simulink model "tennode_3"  (R2018b)
settings: Solver=ode3  StartTime=0.0  StopTime=5  FixedStep=Ts  RelTol=1e-3
values from neighbouring files (symbols this model uses):
  BESS_mode = 0    [load_vars.m]
  line1 = line1_length*R1    (= 0.01273)    [load_vars.m]
  line10 = line10_length*R1    (= 0.01273)    [load_vars.m]
  LINE10_en = 1    [load_vars.m]
  line11 = line11_length*R1    (= 0.01273)    [load_vars.m]
  LINE11_en = 1    [load_vars.m]
  line12 = line12_length*R1    (= 0.02546)    [load_vars.m]
  LINE12_en = 1    [load_vars.m]
  line13 = line13_length*R1    (= 0.015276)    [load_vars.m]
  LINE13_en = 1    [load_vars.m]
  line14 = line14_length*R1    (= 0.019095)    [load_vars.m]
  LINE14_en = 1    [load_vars.m]
  line15 = line15_length*R1    (= 0.014003)    [load_vars.m]
  LINE15_en = 1    [load_vars.m]
  line16 = line16_length*R1    (= 0.034371)    [load_vars.m]
  LINE16_en = 1    [load_vars.m]
  line17 = line17_length*R1    (= 0.017822)    [load_vars.m]
  LINE17_en = 1    [load_vars.m]
  LINE1_en = 1    [load_vars.m]
  line2 = line2_length*R1    (= 0.02546)    [load_vars.m]
  LINE2_en = 1    [load_vars.m]
  line3 = line3_length*R1    (= 0.015276)    [load_vars.m]
  LINE3_en = 1    [load_vars.m]
  line4 = line4_length*R1    (= 0.019095)    [load_vars.m]
  LINE4_en = 1    [load_vars.m]
  line5 = line5_length*R1    (= 0.014003)    [load_vars.m]
  LINE5_en = 1    [load_vars.m]
  line6 = line6_length*R1    (= 0.01273)    [load_vars.m]
  LINE6_en = 1    [load_vars.m]
  line7 = line7_length*R1    (= 0.03819)    [load_vars.m]
  LINE7_en = 1    [load_vars.m]
  line8 = line8_length*R1    (= 0.01273)    [load_vars.m]
  LINE8_en = 1    [load_vars.m]
  line9 = line9_length*R1    (= 0.01273)    [load_vars.m]
  LINE9_en = 1    [load_vars.m]
  t_contingency = 1    [load_vars.m]
  Ts = 0.0001    [load_vars.m]
  uDemand1 = 20e3    (= 20000)    [load_vars.m]
  uDemand10 = 20e3    (= 20000)    [load_vars.m]
  uDemand2 = 20e3    (= 20000)    [load_vars.m]
  uDemand3 = 20e3    (= 20000)    [load_vars.m]
  uDemand4 = 20e3    (= 20000)    [load_vars.m]
  uDemand5 = 20e3    (= 20000)    [load_vars.m]
  uDemand6 = 20e3    (= 20000)    [load_vars.m]
  uDemand7 = 20e3    (= 20000)    [load_vars.m]
  uDemand8 = 20e3    (= 20000)    [load_vars.m]
  uDemand9 = 20e3    (= 20000)    [load_vars.m]
undefined symbols (not defined in the file or in its folder): DER10_BESS_en, DER1_BESS_en, DER2_BESS_en, DER3_BESS_en, DER4_BESS_en, DER5_BESS_en, DER6_BESS_en, DER7_BESS_en, DER8_BESS_en, DER9_BESS_en, DR_capacity_1, DR_capacity_10, DR_capacity_2, DR_capacity_3, DR_capacity_4, DR_capacity_5, DR_capacity_6, DR_capacity_7, DR_capacity_8, DR_capacity_9, P_set1, P_set10, P_set2, P_set3, P_set4, P_set5, P_set6, P_set7, P_set8, P_set9, PV_capacity_1, PV_capacity_10, PV_capacity_2, PV_capacity_3, PV_capacity_4, PV_capacity_5, PV_capacity_6, PV_capacity_7, PV_capacity_8, PV_capacity_9, PV_en_1, PV_en_10, PV_en_2, PV_en_3, PV_en_4, PV_en_5, PV_en_6, PV_en_7, PV_en_8, PV_en_9
libraries: powerlib x232, simulink x66, powerlib_meascontrol x23, sps_avr x1, spsDieselMotorModel x1
(part 4 of 7)

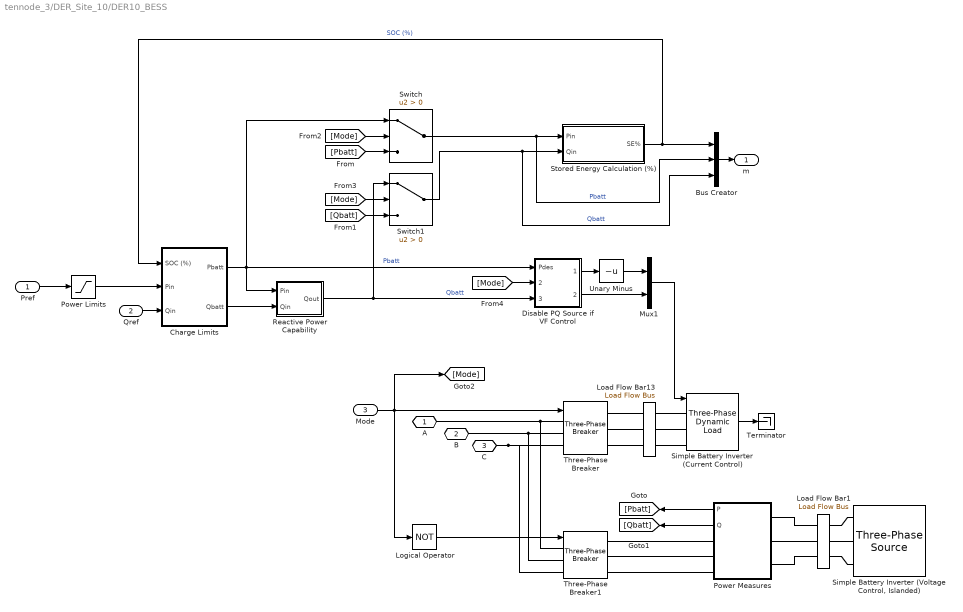
== system tennode_3/DER_Site_10/DER10_BESS ==
  Pref : Inport
  Qref : Inport  Port=2
  Mode : Inport  Port=3
  Bus Creator : BusCreator  Inputs=3
  Charge Limits : Subsystem
  Disable PQ Source if VF Control : Subsystem
  Load Flow Bar1 : powerlib/Measurements/Load Flow Bus  LConnTagsString=a|b|c  RConnTagsString=a|b|c  Phases=ABC  Connectors=on both sides  ID=5  Vbase=400/sqrt(3)  Vref=[1.0 1.0 1.0]  Vangle=[0 -120 120]  VLF=0.9823  VLFb=1.055  VLFc=0.9746  angleLF=-5.476  angleLFb=-122.5  angleLFc=116
      settings: AttributesFormatString=%<ID>  SourceProductName=Simscape Power Systems
  Load Flow Bar13 : powerlib/Measurements/Load Flow Bus  LConnTagsString=a|b|c  RConnTagsString=a|b|c  Phases=ABC  Connectors=on both sides  ID=4  Vbase=400/sqrt(3)  Vref=[1.0 1.0 1.0]  Vangle=[0 -120 120]  VLF=0.9823  VLFb=1.055  VLFc=0.9746  angleLF=-5.476  angleLFb=-122.5  angleLFc=116
      settings: AttributesFormatString=%<ID>  SourceProductName=Simscape Power Systems
  Logical Operator : Logic  Operator=NOT  AllPortsSameDT=off  OutDataTypeStr=boolean
  Mux1 : Mux  Inputs=2
  Power Limits : Saturate  UpperLimit=Pnom  LowerLimit=-Pnom
  Power Measures : Subsystem  VariantControlMode=Label  Variant=on  LabelModeActiveChoice=EMT
  Reactive Power Capability : Subsystem
  Simple Battery Inverter (Current Control) : powerlib/Elements/Three-Phase Dynamic Load  NominalVoltage=[Vn Fn]  ActiveReactivePowers=[-5000 -3.38813e-13]  PositiveSequence=[0.999844 -0.0038635]  ExternalControl=on  NpNq=[1.3 2]  TimeConstants="[0  0  0  0]"  MinimumVoltage=0.7  Tfilter=1e-2  LoadFlowParameters=[4,0,0,0,0]
      settings: SourceProductName=Simscape Electrical  SourceProductBaseCode=PS
  "Simple Battery Inverter (Voltage Control, Islanded)" : powerlib/Electrical Sources/Three-Phase Source  InternalConnection=Yg  VoltagePhases=off  Voltage=Vn  PhaseAngle=0  Voltage_phases=[25e3 25e3 25e3]/sqrt(3)  PhaseAngles_phases=[0 -120 +120]  Frequency=Fn  NonIdealSource=off  SpecifyImpedance=off  Resistance=0.8929  Inductance=16.58e-3  ShortCircuitLevel=100e6  BaseVoltage=25e3  XRratio=7  BusType=swing  Pref=10e3  Qref=0  Prefabc=[10e3, 10e3, 10e3]  Qrefabc=[0, 0, 0]  Qmin=-inf  Qmax=inf
      settings: SourceProductName=Simscape Electrical
  Stored Energy Calculation (%) : Subsystem
  Switch : Switch  Criteria=u2 > Threshold
  Switch1 : Switch  Criteria=u2 > Threshold
  Terminator : Terminator
  Three-Phase Breaker : powerlib/Elements/Three-Phase Breaker  InitialState=closed  SwitchA=on  SwitchB=on  SwitchC=on  SwitchTimes="[1/60  5/60]"  External=on  BreakerResistance=0.01  SnubberResistance=1e6  SnubberCapacitance=inf  Measurements=None
      settings: SourceProductName=Simscape Electrical
  Three-Phase Breaker1 : powerlib/Elements/Three-Phase Breaker  InitialState=open  SwitchA=on  SwitchB=on  SwitchC=on  SwitchTimes="[1/60  5/60]"  External=on  BreakerResistance=0.01  SnubberResistance=1e6  SnubberCapacitance=inf  Measurements=None
      settings: SourceProductName=Simscape Electrical
  Unary Minus : UnaryMinus
  A : PMIOPort  Side=Right
  B : PMIOPort  Port=2  Side=Right
  C : PMIOPort  Port=3  Side=Right
  m : Outport
  wires:
  Disable PQ Source if VF Control/2(Qbatt) -> Mux1/2
  Disable PQ Source if VF Control/1(Pbatt) -> Unary Minus/1
  Reactive Power Capability/1(Qout) -> Switch1/1, Disable PQ Source if VF Control/3(Qdes)  "Qbatt"
  [Mode] -> Disable PQ Source if VF Control/2(Mode)
  Charge Limits/1(Pbatt) -> Disable PQ Source if VF Control/1(Pdes), Reactive Power Capability/1(Pin), Switch/1  "Pbatt"
  [Pbatt] -> Switch/3
  [Qbatt] -> Switch1/3
  [Mode] -> Switch1/2
  [Mode] -> Switch/2
  Switch1/1 -> Stored Energy Calculation (%)/2(Qin), Bus Creator/3  "Qbatt"
  Switch/1 -> Stored Energy Calculation (%)/1(Pin), Bus Creator/2  "Pbatt"
  Power Measures/2(Q) -> [Qbatt]
  Power Measures/1(P) -> [Pbatt]
  Mode/1 -> Three-Phase Breaker/1, Logical Operator/1, [Mode]
  Logical Operator/1 -> Three-Phase Breaker1/1
  Unary Minus/1 -> Mux1/1
  Mux1/1 -> Simple Battery Inverter (Current Control)/1
  Simple Battery Inverter (Current Control)/1 -> Terminator/1
  Pref/1 -> Power Limits/1
  Bus Creator/1 -> m/1
  Stored Energy Calculation (%)/1(SE%) -> Charge Limits/1(SOC (%)), Bus Creator/1  "SOC (%)"
  Power Limits/1 -> Charge Limits/2(Pin)
  Qref/1 -> Charge Limits/3(Qin)
  Charge Limits/2(Qbatt) -> Reactive Power Capability/2(Qin)
  connections:
  Power Measures/RConn3 -- Three-Phase Breaker1/RConn3
  Power Measures/RConn2 -- Three-Phase Breaker1/RConn2
  Power Measures/RConn1 -- Three-Phase Breaker1/RConn1
  Three-Phase Breaker1/LConn1 -- A/RConn1 -- Three-Phase Breaker/LConn1
  Three-Phase Breaker1/LConn2 -- B/RConn1 -- Three-Phase Breaker/LConn2
  C/RConn1 -- Three-Phase Breaker1/LConn3 -- Three-Phase Breaker/LConn3
  Load Flow Bar13/RConn1 -- Three-Phase Breaker/RConn1
  Load Flow Bar13/RConn2 -- Three-Phase Breaker/RConn2
  Load Flow Bar13/RConn3 -- Three-Phase Breaker/RConn3
  Load Flow Bar13/LConn1 -- Simple Battery Inverter (Current Control)/LConn1
  Load Flow Bar13/LConn2 -- Simple Battery Inverter (Current Control)/LConn2
  Load Flow Bar13/LConn3 -- Simple Battery Inverter (Current Control)/LConn3
  "Simple Battery Inverter (Voltage Control, Islanded)"/RConn2 -- Load Flow Bar1/LConn2
  Load Flow Bar1/LConn3 -- "Simple Battery Inverter (Voltage Control, Islanded)"/RConn3
  Load Flow Bar1/LConn1 -- "Simple Battery Inverter (Voltage Control, Islanded)"/RConn1
  Power Measures/LConn1 -- Load Flow Bar1/RConn1
  Power Measures/LConn2 -- Load Flow Bar1/RConn2
  Power Measures/LConn3 -- Load Flow Bar1/RConn3

== system tennode_3/DER_Site_10/DER10_PV  ==
  P : Inport
  Bus Selector : BusSelector  OutputSignals=Active power P (W)
  Constant11 : Constant  Value=0
  Mux1 : Mux  Inputs=2
  Simple Solar Inverter : powerlib/Elements/Three-Phase Dynamic Load  NominalVoltage=[Vn Fn]  ActiveReactivePowers=[-4000 -3.38813e-13]  PositiveSequence=[0.999844 -0.0038635]  ExternalControl=on  NpNq=[1.3 2]  TimeConstants="[0  0  0  0]"  MinimumVoltage=0.7  Tfilter=1e-2  LoadFlowParameters=[4,0,0,0,0]
      settings: SourceProductName=Simscape Electrical  SourceProductBaseCode=PS
  Unary Minus : UnaryMinus
  Unary Minus1 : UnaryMinus
  A : PMIOPort  Side=Right
  B : PMIOPort  Port=2  Side=Right
  C : PMIOPort  Port=3  Side=Right
  m : Outport
  wires:
  P/1 -> Unary Minus/1
  Unary Minus/1 -> Mux1/1
  Mux1/1 -> Simple Solar Inverter/1
  Constant11/1 -> Mux1/2
  Simple Solar Inverter/1 -> Bus Selector/1
  Bus Selector/1 -> Unary Minus1/1  "<Active power P (W)>"
  Unary Minus1/1 -> m/1
  connections:
  Simple Solar Inverter/LConn2 -- B/RConn1
  Simple Solar Inverter/LConn3 -- C/RConn1
  Simple Solar Inverter/LConn1 -- A/RConn1

== system tennode_3/DER_Site_10/Site Load ==
  Load : Inport
  Dynamic Load Control : Subsystem
  Simple Three-Phase Load : powerlib/Elements/Three-Phase Dynamic Load  NominalVoltage=[Vn Fn]  ActiveReactivePowers=[200000 45883.1]  PositiveSequence=[0.999844 -0.0038635]  ExternalControl=on  NpNq=[1.3 2]  TimeConstants="[0  0  0  0]"  MinimumVoltage=0.7  Tfilter=1e-2  LoadFlowParameters=[4,0,0,0,0]
      settings: SourceProductName=Simscape Electrical  SourceProductBaseCode=PS
  A : PMIOPort  Side=Right
  B : PMIOPort  Port=2  Side=Right
  C : PMIOPort  Port=3  Side=Right
  m : Outport
  wires:
  Load/1 -> Dynamic Load Control/1(P0)
  Dynamic Load Control/1(PQ) -> Simple Three-Phase Load/1
  Simple Three-Phase Load/1 -> m/1
  connections:
  Simple Three-Phase Load/LConn1 -- A/RConn1
  Simple Three-Phase Load/LConn3 -- C/RConn1
  Simple Three-Phase Load/LConn2 -- B/RConn1

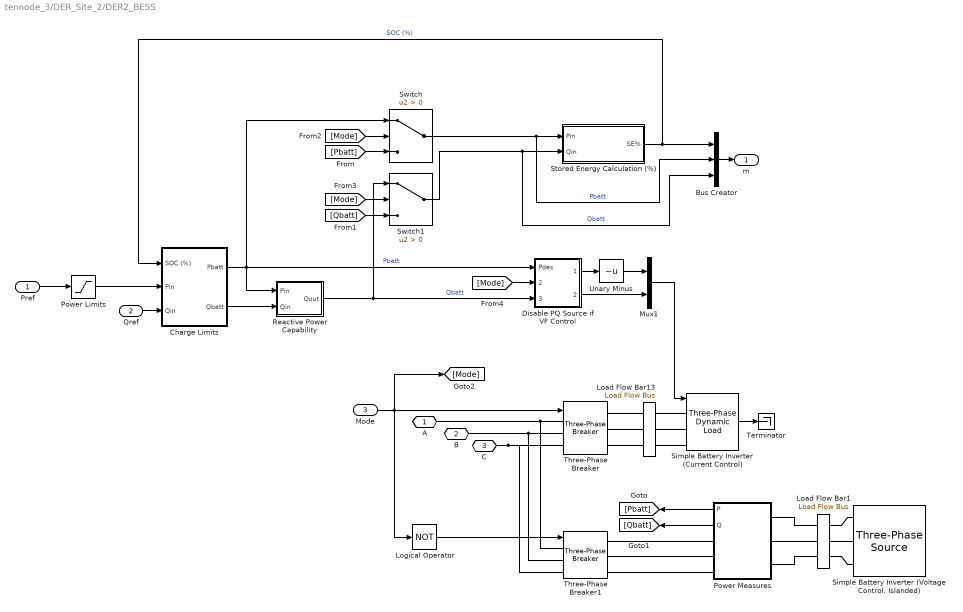
== system tennode_3/DER_Site_2/DER2_BESS ==
  Pref : Inport
  Qref : Inport  Port=2
  Mode : Inport  Port=3
  Bus Creator : BusCreator  Inputs=3
  Charge Limits : Subsystem
  Disable PQ Source if VF Control : Subsystem
  Load Flow Bar1 : powerlib/Measurements/Load Flow Bus  LConnTagsString=a|b|c  RConnTagsString=a|b|c  Phases=ABC  Connectors=on both sides  ID=5  Vbase=400/sqrt(3)  Vref=[1.0 1.0 1.0]  Vangle=[0 -120 120]  VLF=0.9823  VLFb=1.055  VLFc=0.9746  angleLF=-5.476  angleLFb=-122.5  angleLFc=116
      settings: AttributesFormatString=%<ID>  SourceProductName=Simscape Power Systems
  Load Flow Bar13 : powerlib/Measurements/Load Flow Bus  LConnTagsString=a|b|c  RConnTagsString=a|b|c  Phases=ABC  Connectors=on both sides  ID=4  Vbase=400/sqrt(3)  Vref=[1.0 1.0 1.0]  Vangle=[0 -120 120]  VLF=0.9823  VLFb=1.055  VLFc=0.9746  angleLF=-5.476  angleLFb=-122.5  angleLFc=116
      settings: AttributesFormatString=%<ID>  SourceProductName=Simscape Power Systems
  Logical Operator : Logic  Operator=NOT  AllPortsSameDT=off  OutDataTypeStr=boolean
  Mux1 : Mux  Inputs=2
  Power Limits : Saturate  UpperLimit=Pnom  LowerLimit=-Pnom
  Power Measures : Subsystem  VariantControlMode=Label  Variant=on  LabelModeActiveChoice=EMT
  Reactive Power Capability : Subsystem
  Simple Battery Inverter (Current Control) : powerlib/Elements/Three-Phase Dynamic Load  NominalVoltage=[Vn Fn]  ActiveReactivePowers=[-5000 -3.38813e-13]  PositiveSequence=[0.999844 -0.0038635]  ExternalControl=on  NpNq=[1.3 2]  TimeConstants="[0  0  0  0]"  MinimumVoltage=0.7  Tfilter=1e-2  LoadFlowParameters=[4,0,0,0,0]
      settings: SourceProductName=Simscape Electrical  SourceProductBaseCode=PS
  "Simple Battery Inverter (Voltage Control, Islanded)" : powerlib/Electrical Sources/Three-Phase Source  InternalConnection=Yg  VoltagePhases=off  Voltage=Vn  PhaseAngle=0  Voltage_phases=[25e3 25e3 25e3]/sqrt(3)  PhaseAngles_phases=[0 -120 +120]  Frequency=Fn  NonIdealSource=off  SpecifyImpedance=off  Resistance=0.8929  Inductance=16.58e-3  ShortCircuitLevel=100e6  BaseVoltage=25e3  XRratio=7  BusType=swing  Pref=10e3  Qref=0  Prefabc=[10e3, 10e3, 10e3]  Qrefabc=[0, 0, 0]  Qmin=-inf  Qmax=inf
      settings: SourceProductName=Simscape Electrical
  Stored Energy Calculation (%) : Subsystem
  Switch : Switch  Criteria=u2 > Threshold
  Switch1 : Switch  Criteria=u2 > Threshold
  Terminator : Terminator
  Three-Phase Breaker : powerlib/Elements/Three-Phase Breaker  InitialState=closed  SwitchA=on  SwitchB=on  SwitchC=on  SwitchTimes="[1/60  5/60]"  External=on  BreakerResistance=0.01  SnubberResistance=1e6  SnubberCapacitance=inf  Measurements=None
      settings: SourceProductName=Simscape Electrical
  Three-Phase Breaker1 : powerlib/Elements/Three-Phase Breaker  InitialState=open  SwitchA=on  SwitchB=on  SwitchC=on  SwitchTimes="[1/60  5/60]"  External=on  BreakerResistance=0.01  SnubberResistance=1e6  SnubberCapacitance=inf  Measurements=None
      settings: SourceProductName=Simscape Electrical
  Unary Minus : UnaryMinus
  A : PMIOPort  Side=Right
  B : PMIOPort  Port=2  Side=Right
  C : PMIOPort  Port=3  Side=Right
  m : Outport
  wires:
  Disable PQ Source if VF Control/2(Qbatt) -> Mux1/2
  Disable PQ Source if VF Control/1(Pbatt) -> Unary Minus/1
  Reactive Power Capability/1(Qout) -> Switch1/1, Disable PQ Source if VF Control/3(Qdes)  "Qbatt"
  [Mode] -> Disable PQ Source if VF Control/2(Mode)
  Charge Limits/1(Pbatt) -> Disable PQ Source if VF Control/1(Pdes), Reactive Power Capability/1(Pin), Switch/1  "Pbatt"
  [Pbatt] -> Switch/3
  [Qbatt] -> Switch1/3
  [Mode] -> Switch1/2
  [Mode] -> Switch/2
  Switch1/1 -> Stored Energy Calculation (%)/2(Qin), Bus Creator/3  "Qbatt"
  Switch/1 -> Stored Energy Calculation (%)/1(Pin), Bus Creator/2  "Pbatt"
  Power Measures/2(Q) -> [Qbatt]
  Power Measures/1(P) -> [Pbatt]
  Mode/1 -> Three-Phase Breaker/1, Logical Operator/1, [Mode]
  Logical Operator/1 -> Three-Phase Breaker1/1
  Unary Minus/1 -> Mux1/1
  Mux1/1 -> Simple Battery Inverter (Current Control)/1
  Simple Battery Inverter (Current Control)/1 -> Terminator/1
  Pref/1 -> Power Limits/1
  Bus Creator/1 -> m/1
  Stored Energy Calculation (%)/1(SE%) -> Charge Limits/1(SOC (%)), Bus Creator/1  "SOC (%)"
  Power Limits/1 -> Charge Limits/2(Pin)
  Qref/1 -> Charge Limits/3(Qin)
  Charge Limits/2(Qbatt) -> Reactive Power Capability/2(Qin)
  connections:
  Power Measures/RConn3 -- Three-Phase Breaker1/RConn3
  Power Measures/RConn2 -- Three-Phase Breaker1/RConn2
  Power Measures/RConn1 -- Three-Phase Breaker1/RConn1
  Three-Phase Breaker1/LConn1 -- A/RConn1 -- Three-Phase Breaker/LConn1
  Three-Phase Breaker1/LConn2 -- B/RConn1 -- Three-Phase Breaker/LConn2
  C/RConn1 -- Three-Phase Breaker1/LConn3 -- Three-Phase Breaker/LConn3
  Load Flow Bar13/RConn1 -- Three-Phase Breaker/RConn1
  Load Flow Bar13/RConn2 -- Three-Phase Breaker/RConn2
  Load Flow Bar13/RConn3 -- Three-Phase Breaker/RConn3
  Load Flow Bar13/LConn1 -- Simple Battery Inverter (Current Control)/LConn1
  Load Flow Bar13/LConn2 -- Simple Battery Inverter (Current Control)/LConn2
  Load Flow Bar13/LConn3 -- Simple Battery Inverter (Current Control)/LConn3
  "Simple Battery Inverter (Voltage Control, Islanded)"/RConn2 -- Load Flow Bar1/LConn2
  Load Flow Bar1/LConn3 -- "Simple Battery Inverter (Voltage Control, Islanded)"/RConn3
  Load Flow Bar1/LConn1 -- "Simple Battery Inverter (Voltage Control, Islanded)"/RConn1
  Power Measures/LConn1 -- Load Flow Bar1/RConn1
  Power Measures/LConn2 -- Load Flow Bar1/RConn2
  Power Measures/LConn3 -- Load Flow Bar1/RConn3

== system tennode_3/DER_Site_2/DER2_PV  ==
  P : Inport
  Bus Selector : BusSelector  OutputSignals=Active power P (W)
  Constant11 : Constant  Value=0
  Mux1 : Mux  Inputs=2
  Simple Solar Inverter : powerlib/Elements/Three-Phase Dynamic Load  NominalVoltage=[Vn Fn]  ActiveReactivePowers=[-4000 -3.38813e-13]  PositiveSequence=[0.999844 -0.0038635]  ExternalControl=on  NpNq=[1.3 2]  TimeConstants="[0  0  0  0]"  MinimumVoltage=0.7  Tfilter=1e-2  LoadFlowParameters=[4,0,0,0,0]
      settings: SourceProductName=Simscape Electrical  SourceProductBaseCode=PS
  Unary Minus : UnaryMinus
  Unary Minus1 : UnaryMinus
  A : PMIOPort  Side=Right
  B : PMIOPort  Port=2  Side=Right
  C : PMIOPort  Port=3  Side=Right
  m : Outport
  wires:
  P/1 -> Unary Minus/1
  Unary Minus/1 -> Mux1/1
  Mux1/1 -> Simple Solar Inverter/1
  Constant11/1 -> Mux1/2
  Simple Solar Inverter/1 -> Bus Selector/1
  Bus Selector/1 -> Unary Minus1/1  "<Active power P (W)>"
  Unary Minus1/1 -> m/1
  connections:
  Simple Solar Inverter/LConn2 -- B/RConn1
  Simple Solar Inverter/LConn3 -- C/RConn1
  Simple Solar Inverter/LConn1 -- A/RConn1

== system tennode_3/DER_Site_2/Site Load ==
  Load : Inport
  Dynamic Load Control : Subsystem
  Simple Three-Phase Load : powerlib/Elements/Three-Phase Dynamic Load  NominalVoltage=[Vn Fn]  ActiveReactivePowers=[200000 45883.1]  PositiveSequence=[0.999844 -0.0038635]  ExternalControl=on  NpNq=[1.3 2]  TimeConstants="[0  0  0  0]"  MinimumVoltage=0.7  Tfilter=1e-2  LoadFlowParameters=[4,0,0,0,0]
      settings: SourceProductName=Simscape Electrical  SourceProductBaseCode=PS
  A : PMIOPort  Side=Right
  B : PMIOPort  Port=2  Side=Right
  C : PMIOPort  Port=3  Side=Right
  m : Outport
  wires:
  Load/1 -> Dynamic Load Control/1(P0)
  Dynamic Load Control/1(PQ) -> Simple Three-Phase Load/1
  Simple Three-Phase Load/1 -> m/1
  connections:
  Simple Three-Phase Load/LConn1 -- A/RConn1
  Simple Three-Phase Load/LConn3 -- C/RConn1
  Simple Three-Phase Load/LConn2 -- B/RConn1

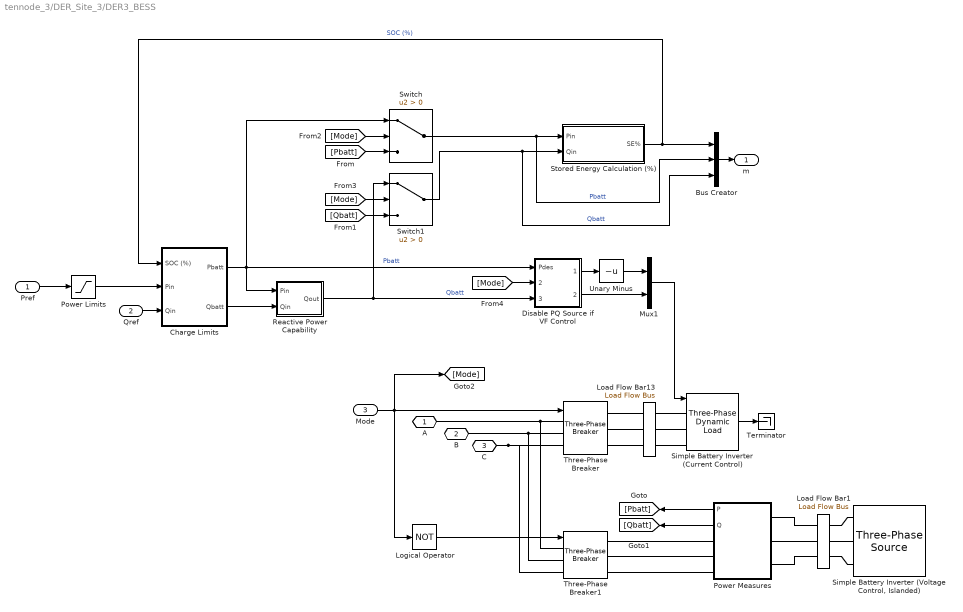
== system tennode_3/DER_Site_3/DER3_BESS ==
  Pref : Inport
  Qref : Inport  Port=2
  Mode : Inport  Port=3
  Bus Creator : BusCreator  Inputs=3
  Charge Limits : Subsystem
  Disable PQ Source if VF Control : Subsystem
  Load Flow Bar1 : powerlib/Measurements/Load Flow Bus  LConnTagsString=a|b|c  RConnTagsString=a|b|c  Phases=ABC  Connectors=on both sides  ID=5  Vbase=400/sqrt(3)  Vref=[1.0 1.0 1.0]  Vangle=[0 -120 120]  VLF=0.9823  VLFb=1.055  VLFc=0.9746  angleLF=-5.476  angleLFb=-122.5  angleLFc=116
      settings: AttributesFormatString=%<ID>  SourceProductName=Simscape Power Systems
  Load Flow Bar13 : powerlib/Measurements/Load Flow Bus  LConnTagsString=a|b|c  RConnTagsString=a|b|c  Phases=ABC  Connectors=on both sides  ID=4  Vbase=400/sqrt(3)  Vref=[1.0 1.0 1.0]  Vangle=[0 -120 120]  VLF=0.9823  VLFb=1.055  VLFc=0.9746  angleLF=-5.476  angleLFb=-122.5  angleLFc=116
      settings: AttributesFormatString=%<ID>  SourceProductName=Simscape Power Systems
  Logical Operator : Logic  Operator=NOT  AllPortsSameDT=off  OutDataTypeStr=boolean
  Mux1 : Mux  Inputs=2
  Power Limits : Saturate  UpperLimit=Pnom  LowerLimit=-Pnom
  Power Measures : Subsystem  VariantControlMode=Label  Variant=on  LabelModeActiveChoice=EMT
  Reactive Power Capability : Subsystem
  Simple Battery Inverter (Current Control) : powerlib/Elements/Three-Phase Dynamic Load  NominalVoltage=[Vn Fn]  ActiveReactivePowers=[-5000 -3.38813e-13]  PositiveSequence=[0.999844 -0.0038635]  ExternalControl=on  NpNq=[1.3 2]  TimeConstants="[0  0  0  0]"  MinimumVoltage=0.7  Tfilter=1e-2  LoadFlowParameters=[4,0,0,0,0]
      settings: SourceProductName=Simscape Electrical  SourceProductBaseCode=PS
  "Simple Battery Inverter (Voltage Control, Islanded)" : powerlib/Electrical Sources/Three-Phase Source  InternalConnection=Yg  VoltagePhases=off  Voltage=Vn  PhaseAngle=0  Voltage_phases=[25e3 25e3 25e3]/sqrt(3)  PhaseAngles_phases=[0 -120 +120]  Frequency=Fn  NonIdealSource=off  SpecifyImpedance=off  Resistance=0.8929  Inductance=16.58e-3  ShortCircuitLevel=100e6  BaseVoltage=25e3  XRratio=7  BusType=swing  Pref=10e3  Qref=0  Prefabc=[10e3, 10e3, 10e3]  Qrefabc=[0, 0, 0]  Qmin=-inf  Qmax=inf
      settings: SourceProductName=Simscape Electrical
  Stored Energy Calculation (%) : Subsystem
  Switch : Switch  Criteria=u2 > Threshold
  Switch1 : Switch  Criteria=u2 > Threshold
  Terminator : Terminator
  Three-Phase Breaker : powerlib/Elements/Three-Phase Breaker  InitialState=closed  SwitchA=on  SwitchB=on  SwitchC=on  SwitchTimes="[1/60  5/60]"  External=on  BreakerResistance=0.01  SnubberResistance=1e6  SnubberCapacitance=inf  Measurements=None
      settings: SourceProductName=Simscape Electrical
  Three-Phase Breaker1 : powerlib/Elements/Three-Phase Breaker  InitialState=open  SwitchA=on  SwitchB=on  SwitchC=on  SwitchTimes="[1/60  5/60]"  External=on  BreakerResistance=0.01  SnubberResistance=1e6  SnubberCapacitance=inf  Measurements=None
      settings: SourceProductName=Simscape Electrical
  Unary Minus : UnaryMinus
  A : PMIOPort  Side=Right
  B : PMIOPort  Port=2  Side=Right
  C : PMIOPort  Port=3  Side=Right
  m : Outport
  wires:
  Disable PQ Source if VF Control/2(Qbatt) -> Mux1/2
  Disable PQ Source if VF Control/1(Pbatt) -> Unary Minus/1
  Reactive Power Capability/1(Qout) -> Switch1/1, Disable PQ Source if VF Control/3(Qdes)  "Qbatt"
  [Mode] -> Disable PQ Source if VF Control/2(Mode)
  Charge Limits/1(Pbatt) -> Disable PQ Source if VF Control/1(Pdes), Reactive Power Capability/1(Pin), Switch/1  "Pbatt"
  [Pbatt] -> Switch/3
  [Qbatt] -> Switch1/3
  [Mode] -> Switch1/2
  [Mode] -> Switch/2
  Switch1/1 -> Stored Energy Calculation (%)/2(Qin), Bus Creator/3  "Qbatt"
  Switch/1 -> Stored Energy Calculation (%)/1(Pin), Bus Creator/2  "Pbatt"
  Power Measures/2(Q) -> [Qbatt]
  Power Measures/1(P) -> [Pbatt]
  Mode/1 -> Three-Phase Breaker/1, Logical Operator/1, [Mode]
  Logical Operator/1 -> Three-Phase Breaker1/1
  Unary Minus/1 -> Mux1/1
  Mux1/1 -> Simple Battery Inverter (Current Control)/1
  Simple Battery Inverter (Current Control)/1 -> Terminator/1
  Pref/1 -> Power Limits/1
  Bus Creator/1 -> m/1
  Stored Energy Calculation (%)/1(SE%) -> Charge Limits/1(SOC (%)), Bus Creator/1  "SOC (%)"
  Power Limits/1 -> Charge Limits/2(Pin)
  Qref/1 -> Charge Limits/3(Qin)
  Charge Limits/2(Qbatt) -> Reactive Power Capability/2(Qin)
  connections:
  Power Measures/RConn3 -- Three-Phase Breaker1/RConn3
  Power Measures/RConn2 -- Three-Phase Breaker1/RConn2
  Power Measures/RConn1 -- Three-Phase Breaker1/RConn1
  Three-Phase Breaker1/LConn1 -- A/RConn1 -- Three-Phase Breaker/LConn1
  Three-Phase Breaker1/LConn2 -- B/RConn1 -- Three-Phase Breaker/LConn2
  C/RConn1 -- Three-Phase Breaker1/LConn3 -- Three-Phase Breaker/LConn3
  Load Flow Bar13/RConn1 -- Three-Phase Breaker/RConn1
  Load Flow Bar13/RConn2 -- Three-Phase Breaker/RConn2
  Load Flow Bar13/RConn3 -- Three-Phase Breaker/RConn3
  Load Flow Bar13/LConn1 -- Simple Battery Inverter (Current Control)/LConn1
  Load Flow Bar13/LConn2 -- Simple Battery Inverter (Current Control)/LConn2
  Load Flow Bar13/LConn3 -- Simple Battery Inverter (Current Control)/LConn3
  "Simple Battery Inverter (Voltage Control, Islanded)"/RConn2 -- Load Flow Bar1/LConn2
  Load Flow Bar1/LConn3 -- "Simple Battery Inverter (Voltage Control, Islanded)"/RConn3
  Load Flow Bar1/LConn1 -- "Simple Battery Inverter (Voltage Control, Islanded)"/RConn1
  Power Measures/LConn1 -- Load Flow Bar1/RConn1
  Power Measures/LConn2 -- Load Flow Bar1/RConn2
  Power Measures/LConn3 -- Load Flow Bar1/RConn3

== system tennode_3/DER_Site_3/DER3_PV  ==
  P : Inport
  Bus Selector : BusSelector  OutputSignals=Active power P (W)
  Constant11 : Constant  Value=0
  Mux1 : Mux  Inputs=2
  Simple Solar Inverter : powerlib/Elements/Three-Phase Dynamic Load  NominalVoltage=[Vn Fn]  ActiveReactivePowers=[-4000 -3.38813e-13]  PositiveSequence=[0.999844 -0.0038635]  ExternalControl=on  NpNq=[1.3 2]  TimeConstants="[0  0  0  0]"  MinimumVoltage=0.7  Tfilter=1e-2  LoadFlowParameters=[4,0,0,0,0]
      settings: SourceProductName=Simscape Electrical  SourceProductBaseCode=PS
  Unary Minus : UnaryMinus
  Unary Minus1 : UnaryMinus
  A : PMIOPort  Side=Right
  B : PMIOPort  Port=2  Side=Right
  C : PMIOPort  Port=3  Side=Right
  m : Outport
  wires:
  P/1 -> Unary Minus/1
  Unary Minus/1 -> Mux1/1
  Mux1/1 -> Simple Solar Inverter/1
  Constant11/1 -> Mux1/2
  Simple Solar Inverter/1 -> Bus Selector/1
  Bus Selector/1 -> Unary Minus1/1  "<Active power P (W)>"
  Unary Minus1/1 -> m/1
  connections:
  Simple Solar Inverter/LConn2 -- B/RConn1
  Simple Solar Inverter/LConn3 -- C/RConn1
  Simple Solar Inverter/LConn1 -- A/RConn1

== system tennode_3/DER_Site_3/Site Load ==
  Load : Inport
  Dynamic Load Control : Subsystem
  Simple Three-Phase Load : powerlib/Elements/Three-Phase Dynamic Load  NominalVoltage=[Vn Fn]  ActiveReactivePowers=[200000 45883.1]  PositiveSequence=[0.999844 -0.0038635]  ExternalControl=on  NpNq=[1.3 2]  TimeConstants="[0  0  0  0]"  MinimumVoltage=0.7  Tfilter=1e-2  LoadFlowParameters=[4,0,0,0,0]
      settings: SourceProductName=Simscape Electrical  SourceProductBaseCode=PS
  A : PMIOPort  Side=Right
  B : PMIOPort  Port=2  Side=Right
  C : PMIOPort  Port=3  Side=Right
  m : Outport
  wires:
  Load/1 -> Dynamic Load Control/1(P0)
  Dynamic Load Control/1(PQ) -> Simple Three-Phase Load/1
  Simple Three-Phase Load/1 -> m/1
  connections:
  Simple Three-Phase Load/LConn1 -- A/RConn1
  Simple Three-Phase Load/LConn3 -- C/RConn1
  Simple Three-Phase Load/LConn2 -- B/RConn1

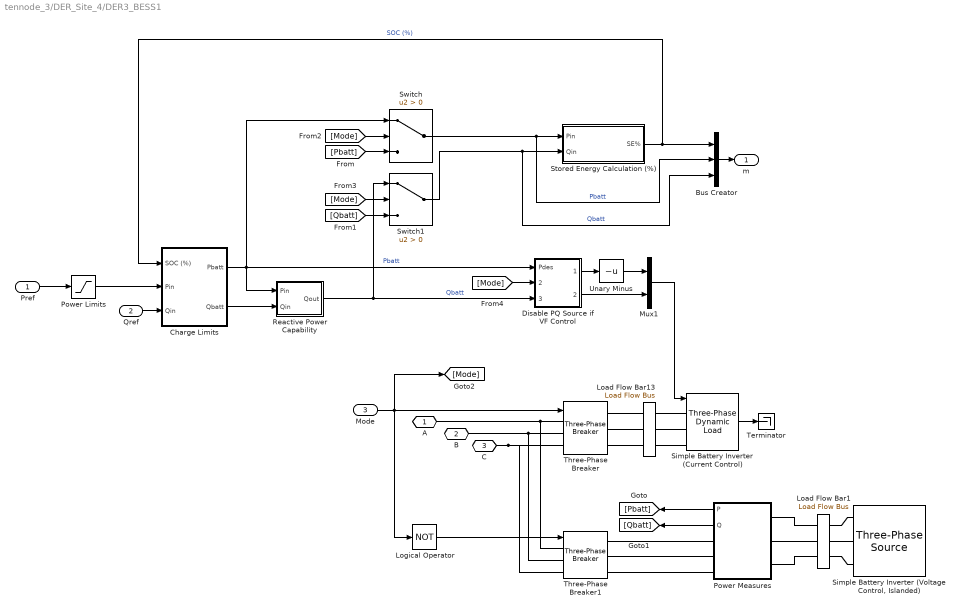
== system tennode_3/DER_Site_4/DER3_BESS1 ==
  Pref : Inport
  Qref : Inport  Port=2
  Mode : Inport  Port=3
  Bus Creator : BusCreator  Inputs=3
  Charge Limits : Subsystem
  Disable PQ Source if VF Control : Subsystem
  Load Flow Bar1 : powerlib/Measurements/Load Flow Bus  LConnTagsString=a|b|c  RConnTagsString=a|b|c  Phases=ABC  Connectors=on both sides  ID=5  Vbase=400/sqrt(3)  Vref=[1.0 1.0 1.0]  Vangle=[0 -120 120]  VLF=0.9823  VLFb=1.055  VLFc=0.9746  angleLF=-5.476  angleLFb=-122.5  angleLFc=116
      settings: AttributesFormatString=%<ID>  SourceProductName=Simscape Power Systems
  Load Flow Bar13 : powerlib/Measurements/Load Flow Bus  LConnTagsString=a|b|c  RConnTagsString=a|b|c  Phases=ABC  Connectors=on both sides  ID=4  Vbase=400/sqrt(3)  Vref=[1.0 1.0 1.0]  Vangle=[0 -120 120]  VLF=0.9823  VLFb=1.055  VLFc=0.9746  angleLF=-5.476  angleLFb=-122.5  angleLFc=116
      settings: AttributesFormatString=%<ID>  SourceProductName=Simscape Power Systems
  Logical Operator : Logic  Operator=NOT  AllPortsSameDT=off  OutDataTypeStr=boolean
  Mux1 : Mux  Inputs=2
  Power Limits : Saturate  UpperLimit=Pnom  LowerLimit=-Pnom
  Power Measures : Subsystem  VariantControlMode=Label  Variant=on  LabelModeActiveChoice=EMT
  Reactive Power Capability : Subsystem
  Simple Battery Inverter (Current Control) : powerlib/Elements/Three-Phase Dynamic Load  NominalVoltage=[Vn Fn]  ActiveReactivePowers=[-5000 -3.38813e-13]  PositiveSequence=[0.999844 -0.0038635]  ExternalControl=on  NpNq=[1.3 2]  TimeConstants="[0  0  0  0]"  MinimumVoltage=0.7  Tfilter=1e-2  LoadFlowParameters=[4,0,0,0,0]
      settings: SourceProductName=Simscape Electrical  SourceProductBaseCode=PS
  "Simple Battery Inverter (Voltage Control, Islanded)" : powerlib/Electrical Sources/Three-Phase Source  InternalConnection=Yg  VoltagePhases=off  Voltage=Vn  PhaseAngle=0  Voltage_phases=[25e3 25e3 25e3]/sqrt(3)  PhaseAngles_phases=[0 -120 +120]  Frequency=Fn  NonIdealSource=off  SpecifyImpedance=off  Resistance=0.8929  Inductance=16.58e-3  ShortCircuitLevel=100e6  BaseVoltage=25e3  XRratio=7  BusType=swing  Pref=10e3  Qref=0  Prefabc=[10e3, 10e3, 10e3]  Qrefabc=[0, 0, 0]  Qmin=-inf  Qmax=inf
      settings: SourceProductName=Simscape Electrical
  Stored Energy Calculation (%) : Subsystem
  Switch : Switch  Criteria=u2 > Threshold
  Switch1 : Switch  Criteria=u2 > Threshold
  Terminator : Terminator
  Three-Phase Breaker : powerlib/Elements/Three-Phase Breaker  InitialState=closed  SwitchA=on  SwitchB=on  SwitchC=on  SwitchTimes="[1/60  5/60]"  External=on  BreakerResistance=0.01  SnubberResistance=1e6  SnubberCapacitance=inf  Measurements=None
      settings: SourceProductName=Simscape Electrical
  Three-Phase Breaker1 : powerlib/Elements/Three-Phase Breaker  InitialState=open  SwitchA=on  SwitchB=on  SwitchC=on  SwitchTimes="[1/60  5/60]"  External=on  BreakerResistance=0.01  SnubberResistance=1e6  SnubberCapacitance=inf  Measurements=None
      settings: SourceProductName=Simscape Electrical
  Unary Minus : UnaryMinus
  A : PMIOPort  Side=Right
  B : PMIOPort  Port=2  Side=Right
  C : PMIOPort  Port=3  Side=Right
  m : Outport
  wires:
  Disable PQ Source if VF Control/2(Qbatt) -> Mux1/2
  Disable PQ Source if VF Control/1(Pbatt) -> Unary Minus/1
  Reactive Power Capability/1(Qout) -> Switch1/1, Disable PQ Source if VF Control/3(Qdes)  "Qbatt"
  [Mode] -> Disable PQ Source if VF Control/2(Mode)
  Charge Limits/1(Pbatt) -> Disable PQ Source if VF Control/1(Pdes), Reactive Power Capability/1(Pin), Switch/1  "Pbatt"
  [Pbatt] -> Switch/3
  [Qbatt] -> Switch1/3
  [Mode] -> Switch1/2
  [Mode] -> Switch/2
  Switch1/1 -> Stored Energy Calculation (%)/2(Qin), Bus Creator/3  "Qbatt"
  Switch/1 -> Stored Energy Calculation (%)/1(Pin), Bus Creator/2  "Pbatt"
  Power Measures/2(Q) -> [Qbatt]
  Power Measures/1(P) -> [Pbatt]
  Mode/1 -> Three-Phase Breaker/1, Logical Operator/1, [Mode]
  Logical Operator/1 -> Three-Phase Breaker1/1
  Unary Minus/1 -> Mux1/1
  Mux1/1 -> Simple Battery Inverter (Current Control)/1
  Simple Battery Inverter (Current Control)/1 -> Terminator/1
  Pref/1 -> Power Limits/1
  Bus Creator/1 -> m/1
  Stored Energy Calculation (%)/1(SE%) -> Charge Limits/1(SOC (%)), Bus Creator/1  "SOC (%)"
  Power Limits/1 -> Charge Limits/2(Pin)
  Qref/1 -> Charge Limits/3(Qin)
  Charge Limits/2(Qbatt) -> Reactive Power Capability/2(Qin)
  connections:
  Power Measures/RConn3 -- Three-Phase Breaker1/RConn3
  Power Measures/RConn2 -- Three-Phase Breaker1/RConn2
  Power Measures/RConn1 -- Three-Phase Breaker1/RConn1
  Three-Phase Breaker1/LConn1 -- A/RConn1 -- Three-Phase Breaker/LConn1
  Three-Phase Breaker1/LConn2 -- B/RConn1 -- Three-Phase Breaker/LConn2
  C/RConn1 -- Three-Phase Breaker1/LConn3 -- Three-Phase Breaker/LConn3
  Load Flow Bar13/RConn1 -- Three-Phase Breaker/RConn1
  Load Flow Bar13/RConn2 -- Three-Phase Breaker/RConn2
  Load Flow Bar13/RConn3 -- Three-Phase Breaker/RConn3
  Load Flow Bar13/LConn1 -- Simple Battery Inverter (Current Control)/LConn1
  Load Flow Bar13/LConn2 -- Simple Battery Inverter (Current Control)/LConn2
  Load Flow Bar13/LConn3 -- Simple Battery Inverter (Current Control)/LConn3
  "Simple Battery Inverter (Voltage Control, Islanded)"/RConn2 -- Load Flow Bar1/LConn2
  Load Flow Bar1/LConn3 -- "Simple Battery Inverter (Voltage Control, Islanded)"/RConn3
  Load Flow Bar1/LConn1 -- "Simple Battery Inverter (Voltage Control, Islanded)"/RConn1
  Power Measures/LConn1 -- Load Flow Bar1/RConn1
  Power Measures/LConn2 -- Load Flow Bar1/RConn2
  Power Measures/LConn3 -- Load Flow Bar1/RConn3

== system tennode_3/DER_Site_4/DER3_PV  ==
  P : Inport
  Bus Selector : BusSelector  OutputSignals=Active power P (W)
  Constant11 : Constant  Value=0
  Mux1 : Mux  Inputs=2
  Simple Solar Inverter : powerlib/Elements/Three-Phase Dynamic Load  NominalVoltage=[Vn Fn]  ActiveReactivePowers=[-4000 -3.38813e-13]  PositiveSequence=[0.999844 -0.0038635]  ExternalControl=on  NpNq=[1.3 2]  TimeConstants="[0  0  0  0]"  MinimumVoltage=0.7  Tfilter=1e-2  LoadFlowParameters=[4,0,0,0,0]
      settings: SourceProductName=Simscape Electrical  SourceProductBaseCode=PS
  Unary Minus : UnaryMinus
  Unary Minus1 : UnaryMinus
  A : PMIOPort  Side=Right
  B : PMIOPort  Port=2  Side=Right
  C : PMIOPort  Port=3  Side=Right
  m : Outport
  wires:
  P/1 -> Unary Minus/1
  Unary Minus/1 -> Mux1/1
  Mux1/1 -> Simple Solar Inverter/1
  Constant11/1 -> Mux1/2
  Simple Solar Inverter/1 -> Bus Selector/1
  Bus Selector/1 -> Unary Minus1/1  "<Active power P (W)>"
  Unary Minus1/1 -> m/1
  connections:
  Simple Solar Inverter/LConn2 -- B/RConn1
  Simple Solar Inverter/LConn3 -- C/RConn1
  Simple Solar Inverter/LConn1 -- A/RConn1

== system tennode_3/DER_Site_4/Site Load ==
  Load : Inport
  Dynamic Load Control : Subsystem
  Simple Three-Phase Load : powerlib/Elements/Three-Phase Dynamic Load  NominalVoltage=[Vn Fn]  ActiveReactivePowers=[200000 45883.1]  PositiveSequence=[0.999844 -0.0038635]  ExternalControl=on  NpNq=[1.3 2]  TimeConstants="[0  0  0  0]"  MinimumVoltage=0.7  Tfilter=1e-2  LoadFlowParameters=[4,0,0,0,0]
      settings: SourceProductName=Simscape Electrical  SourceProductBaseCode=PS
  A : PMIOPort  Side=Right
  B : PMIOPort  Port=2  Side=Right
  C : PMIOPort  Port=3  Side=Right
  m : Outport
  wires:
  Load/1 -> Dynamic Load Control/1(P0)
  Dynamic Load Control/1(PQ) -> Simple Three-Phase Load/1
  Simple Three-Phase Load/1 -> m/1
  connections:
  Simple Three-Phase Load/LConn1 -- A/RConn1
  Simple Three-Phase Load/LConn3 -- C/RConn1
  Simple Three-Phase Load/LConn2 -- B/RConn1

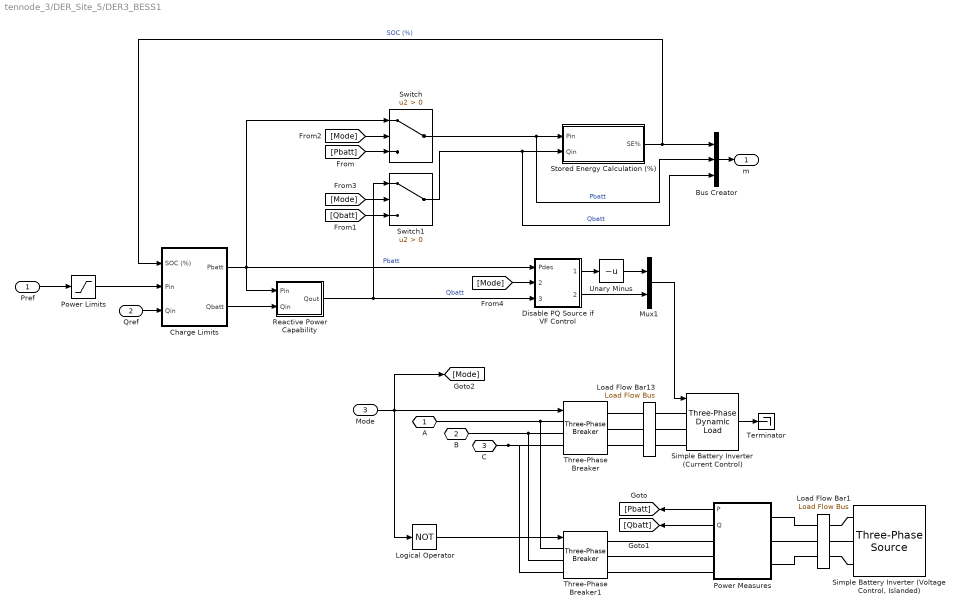
== system tennode_3/DER_Site_5/DER3_BESS1 ==
  Pref : Inport
  Qref : Inport  Port=2
  Mode : Inport  Port=3
  Bus Creator : BusCreator  Inputs=3
  Charge Limits : Subsystem
  Disable PQ Source if VF Control : Subsystem
  Load Flow Bar1 : powerlib/Measurements/Load Flow Bus  LConnTagsString=a|b|c  RConnTagsString=a|b|c  Phases=ABC  Connectors=on both sides  ID=5  Vbase=400/sqrt(3)  Vref=[1.0 1.0 1.0]  Vangle=[0 -120 120]  VLF=0.9823  VLFb=1.055  VLFc=0.9746  angleLF=-5.476  angleLFb=-122.5  angleLFc=116
      settings: AttributesFormatString=%<ID>  SourceProductName=Simscape Power Systems
  Load Flow Bar13 : powerlib/Measurements/Load Flow Bus  LConnTagsString=a|b|c  RConnTagsString=a|b|c  Phases=ABC  Connectors=on both sides  ID=4  Vbase=400/sqrt(3)  Vref=[1.0 1.0 1.0]  Vangle=[0 -120 120]  VLF=0.9823  VLFb=1.055  VLFc=0.9746  angleLF=-5.476  angleLFb=-122.5  angleLFc=116
      settings: AttributesFormatString=%<ID>  SourceProductName=Simscape Power Systems
  Logical Operator : Logic  Operator=NOT  AllPortsSameDT=off  OutDataTypeStr=boolean
  Mux1 : Mux  Inputs=2
  Power Limits : Saturate  UpperLimit=Pnom  LowerLimit=-Pnom
  Power Measures : Subsystem  VariantControlMode=Label  Variant=on  LabelModeActiveChoice=EMT
  Reactive Power Capability : Subsystem
  Simple Battery Inverter (Current Control) : powerlib/Elements/Three-Phase Dynamic Load  NominalVoltage=[Vn Fn]  ActiveReactivePowers=[-5000 -3.38813e-13]  PositiveSequence=[0.999844 -0.0038635]  ExternalControl=on  NpNq=[1.3 2]  TimeConstants="[0  0  0  0]"  MinimumVoltage=0.7  Tfilter=1e-2  LoadFlowParameters=[4,0,0,0,0]
      settings: SourceProductName=Simscape Electrical  SourceProductBaseCode=PS
  "Simple Battery Inverter (Voltage Control, Islanded)" : powerlib/Electrical Sources/Three-Phase Source  InternalConnection=Yg  VoltagePhases=off  Voltage=Vn  PhaseAngle=0  Voltage_phases=[25e3 25e3 25e3]/sqrt(3)  PhaseAngles_phases=[0 -120 +120]  Frequency=Fn  NonIdealSource=off  SpecifyImpedance=off  Resistance=0.8929  Inductance=16.58e-3  ShortCircuitLevel=100e6  BaseVoltage=25e3  XRratio=7  BusType=swing  Pref=10e3  Qref=0  Prefabc=[10e3, 10e3, 10e3]  Qrefabc=[0, 0, 0]  Qmin=-inf  Qmax=inf
      settings: SourceProductName=Simscape Electrical
  Stored Energy Calculation (%) : Subsystem
  Switch : Switch  Criteria=u2 > Threshold
  Switch1 : Switch  Criteria=u2 > Threshold
  Terminator : Terminator
  Three-Phase Breaker : powerlib/Elements/Three-Phase Breaker  InitialState=closed  SwitchA=on  SwitchB=on  SwitchC=on  SwitchTimes="[1/60  5/60]"  External=on  BreakerResistance=0.01  SnubberResistance=1e6  SnubberCapacitance=inf  Measurements=None
      settings: SourceProductName=Simscape Electrical
  Three-Phase Breaker1 : powerlib/Elements/Three-Phase Breaker  InitialState=open  SwitchA=on  SwitchB=on  SwitchC=on  SwitchTimes="[1/60  5/60]"  External=on  BreakerResistance=0.01  SnubberResistance=1e6  SnubberCapacitance=inf  Measurements=None
      settings: SourceProductName=Simscape Electrical
  Unary Minus : UnaryMinus
  A : PMIOPort  Side=Right
  B : PMIOPort  Port=2  Side=Right
  C : PMIOPort  Port=3  Side=Right
  m : Outport
  wires:
  Disable PQ Source if VF Control/2(Qbatt) -> Mux1/2
  Disable PQ Source if VF Control/1(Pbatt) -> Unary Minus/1
  Reactive Power Capability/1(Qout) -> Switch1/1, Disable PQ Source if VF Control/3(Qdes)  "Qbatt"
  [Mode] -> Disable PQ Source if VF Control/2(Mode)
  Charge Limits/1(Pbatt) -> Disable PQ Source if VF Control/1(Pdes), Reactive Power Capability/1(Pin), Switch/1  "Pbatt"
  [Pbatt] -> Switch/3
  [Qbatt] -> Switch1/3
  [Mode] -> Switch1/2
  [Mode] -> Switch/2
  Switch1/1 -> Stored Energy Calculation (%)/2(Qin), Bus Creator/3  "Qbatt"
  Switch/1 -> Stored Energy Calculation (%)/1(Pin), Bus Creator/2  "Pbatt"
  Power Measures/2(Q) -> [Qbatt]
  Power Measures/1(P) -> [Pbatt]
  Mode/1 -> Three-Phase Breaker/1, Logical Operator/1, [Mode]
  Logical Operator/1 -> Three-Phase Breaker1/1
  Unary Minus/1 -> Mux1/1
  Mux1/1 -> Simple Battery Inverter (Current Control)/1
  Simple Battery Inverter (Current Control)/1 -> Terminator/1
  Pref/1 -> Power Limits/1
  Bus Creator/1 -> m/1
  Stored Energy Calculation (%)/1(SE%) -> Charge Limits/1(SOC (%)), Bus Creator/1  "SOC (%)"
  Power Limits/1 -> Charge Limits/2(Pin)
  Qref/1 -> Charge Limits/3(Qin)
  Charge Limits/2(Qbatt) -> Reactive Power Capability/2(Qin)
  connections:
  Power Measures/RConn3 -- Three-Phase Breaker1/RConn3
  Power Measures/RConn2 -- Three-Phase Breaker1/RConn2
  Power Measures/RConn1 -- Three-Phase Breaker1/RConn1
  Three-Phase Breaker1/LConn1 -- A/RConn1 -- Three-Phase Breaker/LConn1
  Three-Phase Breaker1/LConn2 -- B/RConn1 -- Three-Phase Breaker/LConn2
  C/RConn1 -- Three-Phase Breaker1/LConn3 -- Three-Phase Breaker/LConn3
  Load Flow Bar13/RConn1 -- Three-Phase Breaker/RConn1
  Load Flow Bar13/RConn2 -- Three-Phase Breaker/RConn2
  Load Flow Bar13/RConn3 -- Three-Phase Breaker/RConn3
  Load Flow Bar13/LConn1 -- Simple Battery Inverter (Current Control)/LConn1
  Load Flow Bar13/LConn2 -- Simple Battery Inverter (Current Control)/LConn2
  Load Flow Bar13/LConn3 -- Simple Battery Inverter (Current Control)/LConn3
  "Simple Battery Inverter (Voltage Control, Islanded)"/RConn2 -- Load Flow Bar1/LConn2
  Load Flow Bar1/LConn3 -- "Simple Battery Inverter (Voltage Control, Islanded)"/RConn3
  Load Flow Bar1/LConn1 -- "Simple Battery Inverter (Voltage Control, Islanded)"/RConn1
  Power Measures/LConn1 -- Load Flow Bar1/RConn1
  Power Measures/LConn2 -- Load Flow Bar1/RConn2
  Power Measures/LConn3 -- Load Flow Bar1/RConn3

== system tennode_3/DER_Site_5/DER3_PV  ==
  P : Inport
  Bus Selector : BusSelector  OutputSignals=Active power P (W)
  Constant11 : Constant  Value=0
  Mux1 : Mux  Inputs=2
  Simple Solar Inverter : powerlib/Elements/Three-Phase Dynamic Load  NominalVoltage=[Vn Fn]  ActiveReactivePowers=[-4000 -3.38813e-13]  PositiveSequence=[0.999844 -0.0038635]  ExternalControl=on  NpNq=[1.3 2]  TimeConstants="[0  0  0  0]"  MinimumVoltage=0.7  Tfilter=1e-2  LoadFlowParameters=[4,0,0,0,0]
      settings: SourceProductName=Simscape Electrical  SourceProductBaseCode=PS
  Unary Minus : UnaryMinus
  Unary Minus1 : UnaryMinus
  A : PMIOPort  Side=Right
  B : PMIOPort  Port=2  Side=Right
  C : PMIOPort  Port=3  Side=Right
  m : Outport
  wires:
  P/1 -> Unary Minus/1
  Unary Minus/1 -> Mux1/1
  Mux1/1 -> Simple Solar Inverter/1
  Constant11/1 -> Mux1/2
  Simple Solar Inverter/1 -> Bus Selector/1
  Bus Selector/1 -> Unary Minus1/1  "<Active power P (W)>"
  Unary Minus1/1 -> m/1
  connections:
  Simple Solar Inverter/LConn2 -- B/RConn1
  Simple Solar Inverter/LConn3 -- C/RConn1
  Simple Solar Inverter/LConn1 -- A/RConn1

== system tennode_3/DER_Site_5/Site Load ==
  Load : Inport
  Dynamic Load Control : Subsystem
  Simple Three-Phase Load : powerlib/Elements/Three-Phase Dynamic Load  NominalVoltage=[Vn Fn]  ActiveReactivePowers=[200000 45883.1]  PositiveSequence=[0.999844 -0.0038635]  ExternalControl=on  NpNq=[1.3 2]  TimeConstants="[0  0  0  0]"  MinimumVoltage=0.7  Tfilter=1e-2  LoadFlowParameters=[4,0,0,0,0]
      settings: SourceProductName=Simscape Electrical  SourceProductBaseCode=PS
  A : PMIOPort  Side=Right
  B : PMIOPort  Port=2  Side=Right
  C : PMIOPort  Port=3  Side=Right
  m : Outport
  wires:
  Load/1 -> Dynamic Load Control/1(P0)
  Dynamic Load Control/1(PQ) -> Simple Three-Phase Load/1
  Simple Three-Phase Load/1 -> m/1
  connections:
  Simple Three-Phase Load/LConn1 -- A/RConn1
  Simple Three-Phase Load/LConn3 -- C/RConn1
  Simple Three-Phase Load/LConn2 -- B/RConn1

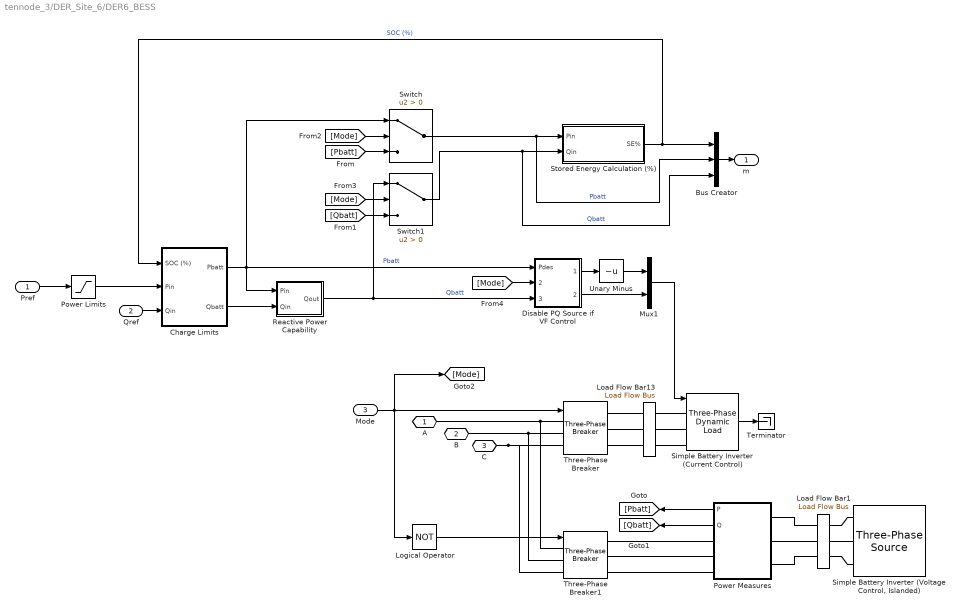
== system tennode_3/DER_Site_6/DER6_BESS ==
  Pref : Inport
  Qref : Inport  Port=2
  Mode : Inport  Port=3
  Bus Creator : BusCreator  Inputs=3
  Charge Limits : Subsystem
  Disable PQ Source if VF Control : Subsystem
  Load Flow Bar1 : powerlib/Measurements/Load Flow Bus  LConnTagsString=a|b|c  RConnTagsString=a|b|c  Phases=ABC  Connectors=on both sides  ID=5  Vbase=400/sqrt(3)  Vref=[1.0 1.0 1.0]  Vangle=[0 -120 120]  VLF=0.9823  VLFb=1.055  VLFc=0.9746  angleLF=-5.476  angleLFb=-122.5  angleLFc=116
      settings: AttributesFormatString=%<ID>  SourceProductName=Simscape Power Systems
  Load Flow Bar13 : powerlib/Measurements/Load Flow Bus  LConnTagsString=a|b|c  RConnTagsString=a|b|c  Phases=ABC  Connectors=on both sides  ID=4  Vbase=400/sqrt(3)  Vref=[1.0 1.0 1.0]  Vangle=[0 -120 120]  VLF=0.9823  VLFb=1.055  VLFc=0.9746  angleLF=-5.476  angleLFb=-122.5  angleLFc=116
      settings: AttributesFormatString=%<ID>  SourceProductName=Simscape Power Systems
  Logical Operator : Logic  Operator=NOT  AllPortsSameDT=off  OutDataTypeStr=boolean
  Mux1 : Mux  Inputs=2
  Power Limits : Saturate  UpperLimit=Pnom  LowerLimit=-Pnom
  Power Measures : Subsystem  VariantControlMode=Label  Variant=on  LabelModeActiveChoice=EMT
  Reactive Power Capability : Subsystem
  Simple Battery Inverter (Current Control) : powerlib/Elements/Three-Phase Dynamic Load  NominalVoltage=[Vn Fn]  ActiveReactivePowers=[-5000 -3.38813e-13]  PositiveSequence=[0.999844 -0.0038635]  ExternalControl=on  NpNq=[1.3 2]  TimeConstants="[0  0  0  0]"  MinimumVoltage=0.7  Tfilter=1e-2  LoadFlowParameters=[4,0,0,0,0]
      settings: SourceProductName=Simscape Electrical  SourceProductBaseCode=PS
  "Simple Battery Inverter (Voltage Control, Islanded)" : powerlib/Electrical Sources/Three-Phase Source  InternalConnection=Yg  VoltagePhases=off  Voltage=Vn  PhaseAngle=0  Voltage_phases=[25e3 25e3 25e3]/sqrt(3)  PhaseAngles_phases=[0 -120 +120]  Frequency=Fn  NonIdealSource=off  SpecifyImpedance=off  Resistance=0.8929  Inductance=16.58e-3  ShortCircuitLevel=100e6  BaseVoltage=25e3  XRratio=7  BusType=swing  Pref=10e3  Qref=0  Prefabc=[10e3, 10e3, 10e3]  Qrefabc=[0, 0, 0]  Qmin=-inf  Qmax=inf
      settings: SourceProductName=Simscape Electrical
  Stored Energy Calculation (%) : Subsystem
  Switch : Switch  Criteria=u2 > Threshold
  Switch1 : Switch  Criteria=u2 > Threshold
  Terminator : Terminator
  Three-Phase Breaker : powerlib/Elements/Three-Phase Breaker  InitialState=closed  SwitchA=on  SwitchB=on  SwitchC=on  SwitchTimes="[1/60  5/60]"  External=on  BreakerResistance=0.01  SnubberResistance=1e6  SnubberCapacitance=inf  Measurements=None
      settings: SourceProductName=Simscape Electrical
  Three-Phase Breaker1 : powerlib/Elements/Three-Phase Breaker  InitialState=open  SwitchA=on  SwitchB=on  SwitchC=on  SwitchTimes="[1/60  5/60]"  External=on  BreakerResistance=0.01  SnubberResistance=1e6  SnubberCapacitance=inf  Measurements=None
      settings: SourceProductName=Simscape Electrical
  Unary Minus : UnaryMinus
  A : PMIOPort  Side=Right
  B : PMIOPort  Port=2  Side=Right
  C : PMIOPort  Port=3  Side=Right
  m : Outport
  wires:
  Disable PQ Source if VF Control/2(Qbatt) -> Mux1/2
  Disable PQ Source if VF Control/1(Pbatt) -> Unary Minus/1
  Reactive Power Capability/1(Qout) -> Switch1/1, Disable PQ Source if VF Control/3(Qdes)  "Qbatt"
  [Mode] -> Disable PQ Source if VF Control/2(Mode)
  Charge Limits/1(Pbatt) -> Disable PQ Source if VF Control/1(Pdes), Reactive Power Capability/1(Pin), Switch/1  "Pbatt"
  [Pbatt] -> Switch/3
  [Qbatt] -> Switch1/3
  [Mode] -> Switch1/2
  [Mode] -> Switch/2
  Switch1/1 -> Stored Energy Calculation (%)/2(Qin), Bus Creator/3  "Qbatt"
  Switch/1 -> Stored Energy Calculation (%)/1(Pin), Bus Creator/2  "Pbatt"
  Power Measures/2(Q) -> [Qbatt]
  Power Measures/1(P) -> [Pbatt]
  Mode/1 -> Three-Phase Breaker/1, Logical Operator/1, [Mode]
  Logical Operator/1 -> Three-Phase Breaker1/1
  Unary Minus/1 -> Mux1/1
  Mux1/1 -> Simple Battery Inverter (Current Control)/1
  Simple Battery Inverter (Current Control)/1 -> Terminator/1
  Pref/1 -> Power Limits/1
  Bus Creator/1 -> m/1
  Stored Energy Calculation (%)/1(SE%) -> Charge Limits/1(SOC (%)), Bus Creator/1  "SOC (%)"
  Power Limits/1 -> Charge Limits/2(Pin)
  Qref/1 -> Charge Limits/3(Qin)
  Charge Limits/2(Qbatt) -> Reactive Power Capability/2(Qin)
  connections:
  Power Measures/RConn3 -- Three-Phase Breaker1/RConn3
  Power Measures/RConn2 -- Three-Phase Breaker1/RConn2
  Power Measures/RConn1 -- Three-Phase Breaker1/RConn1
  Three-Phase Breaker1/LConn1 -- A/RConn1 -- Three-Phase Breaker/LConn1
  Three-Phase Breaker1/LConn2 -- B/RConn1 -- Three-Phase Breaker/LConn2
  C/RConn1 -- Three-Phase Breaker1/LConn3 -- Three-Phase Breaker/LConn3
  Load Flow Bar13/RConn1 -- Three-Phase Breaker/RConn1
  Load Flow Bar13/RConn2 -- Three-Phase Breaker/RConn2
  Load Flow Bar13/RConn3 -- Three-Phase Breaker/RConn3
  Load Flow Bar13/LConn1 -- Simple Battery Inverter (Current Control)/LConn1
  Load Flow Bar13/LConn2 -- Simple Battery Inverter (Current Control)/LConn2
  Load Flow Bar13/LConn3 -- Simple Battery Inverter (Current Control)/LConn3
  "Simple Battery Inverter (Voltage Control, Islanded)"/RConn2 -- Load Flow Bar1/LConn2
  Load Flow Bar1/LConn3 -- "Simple Battery Inverter (Voltage Control, Islanded)"/RConn3
  Load Flow Bar1/LConn1 -- "Simple Battery Inverter (Voltage Control, Islanded)"/RConn1
  Power Measures/LConn1 -- Load Flow Bar1/RConn1
  Power Measures/LConn2 -- Load Flow Bar1/RConn2
  Power Measures/LConn3 -- Load Flow Bar1/RConn3

== system tennode_3/DER_Site_6/DER6_PV  ==
  P : Inport
  Bus Selector : BusSelector  OutputSignals=Active power P (W)
  Constant11 : Constant  Value=0
  Mux1 : Mux  Inputs=2
  Simple Solar Inverter : powerlib/Elements/Three-Phase Dynamic Load  NominalVoltage=[Vn Fn]  ActiveReactivePowers=[-4000 -3.38813e-13]  PositiveSequence=[0.999844 -0.0038635]  ExternalControl=on  NpNq=[1.3 2]  TimeConstants="[0  0  0  0]"  MinimumVoltage=0.7  Tfilter=1e-2  LoadFlowParameters=[4,0,0,0,0]
      settings: SourceProductName=Simscape Electrical  SourceProductBaseCode=PS
  Unary Minus : UnaryMinus
  Unary Minus1 : UnaryMinus
  A : PMIOPort  Side=Right
  B : PMIOPort  Port=2  Side=Right
  C : PMIOPort  Port=3  Side=Right
  m : Outport
  wires:
  P/1 -> Unary Minus/1
  Unary Minus/1 -> Mux1/1
  Mux1/1 -> Simple Solar Inverter/1
  Constant11/1 -> Mux1/2
  Simple Solar Inverter/1 -> Bus Selector/1
  Bus Selector/1 -> Unary Minus1/1  "<Active power P (W)>"
  Unary Minus1/1 -> m/1
  connections:
  Simple Solar Inverter/LConn2 -- B/RConn1
  Simple Solar Inverter/LConn3 -- C/RConn1
  Simple Solar Inverter/LConn1 -- A/RConn1

== system tennode_3/DER_Site_6/Site Load ==
  Load : Inport
  Dynamic Load Control : Subsystem
  Simple Three-Phase Load : powerlib/Elements/Three-Phase Dynamic Load  NominalVoltage=[Vn Fn]  ActiveReactivePowers=[200000 45883.1]  PositiveSequence=[0.999844 -0.0038635]  ExternalControl=on  NpNq=[1.3 2]  TimeConstants="[0  0  0  0]"  MinimumVoltage=0.7  Tfilter=1e-2  LoadFlowParameters=[4,0,0,0,0]
      settings: SourceProductName=Simscape Electrical  SourceProductBaseCode=PS
  A : PMIOPort  Side=Right
  B : PMIOPort  Port=2  Side=Right
  C : PMIOPort  Port=3  Side=Right
  m : Outport
  wires:
  Load/1 -> Dynamic Load Control/1(P0)
  Dynamic Load Control/1(PQ) -> Simple Three-Phase Load/1
  Simple Three-Phase Load/1 -> m/1
  connections:
  Simple Three-Phase Load/LConn1 -- A/RConn1
  Simple Three-Phase Load/LConn3 -- C/RConn1
  Simple Three-Phase Load/LConn2 -- B/RConn1
